simulink model "twoarea_system_test"  (R2014b)
settings: Solver=ode3  StartTime=0.0  StopTime=2  FixedStep=50e-6  RelTol=1e-3
libraries: powerlib x82
settings Model: Creator=saqibhasan  LastModifiedBy=saqibhasan
settings RTWCC: GenCodeOnly=on

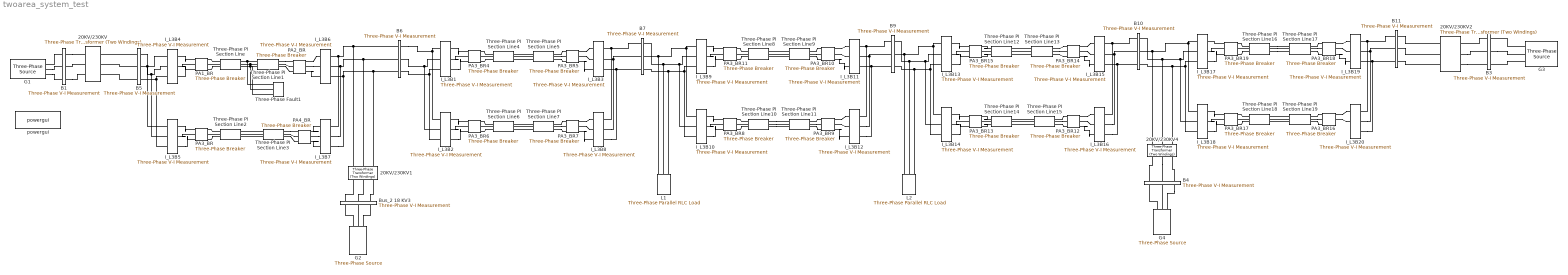
== system twoarea_system_test ==
  20KV/230KV : powerlib/Elements/Three-Phase Transformer (Two Windings)  Winding1Connection=Yg  UNITS=pu  NominalPower=[ 100e6 , 60 ]  Winding1=[ 20e3 , 0 , 3.980e-4]  Winding2Connection=Yg  Winding2=[ 230e3 , 0, 3.980e-4]  SetSaturation=off  Rm=500  Lm=500  Saturation=[ 0,0 ; 0.0024,1.2 ; 1.0,1.52 ]  Hysteresis=off  DataFile='hysteresis'  SetInitialFlux=off  InitialFluxes=[ 0.8 , -0.8 , 0.7 ]  Measurements=None  MoreParameters=off  BreakLoop=off  DataType=off  TransfoNumber=1
  20KV/230KV1 : powerlib/Elements/Three-Phase Transformer (Two Windings)  Winding1Connection=Yg  UNITS=pu  NominalPower=[ 900e6 , 60 ]  Winding1=[ 20e3 , 0 , 3.980e-4]  Winding2Connection=Yg  Winding2=[ 230e3 , 0, 3.980e-4]  SetSaturation=off  Rm=500  Lm=500  Saturation=[ 0,0 ; 0.0024,1.2 ; 1.0,1.52 ]  Hysteresis=off  DataFile='hysteresis'  SetInitialFlux=off  InitialFluxes=[ 0.8 , -0.8 , 0.7 ]  Measurements=None  MoreParameters=off  BreakLoop=off  DataType=off  TransfoNumber=1
  20KV/230KV2 : powerlib/Elements/Three-Phase Transformer (Two Windings)  Winding1Connection=Yg  UNITS=pu  NominalPower=[ 900e6 , 60 ]  Winding1=[ 20e3 , 0 , 3.980e-4]  Winding2Connection=Yg  Winding2=[ 230e3 , 0, 3.980e-4]  SetSaturation=off  Rm=500  Lm=500  Saturation=[ 0,0 ; 0.0024,1.2 ; 1.0,1.52 ]  Hysteresis=off  DataFile='hysteresis'  SetInitialFlux=off  InitialFluxes=[ 0.8 , -0.8 , 0.7 ]  Measurements=None  MoreParameters=off  BreakLoop=off  DataType=off  TransfoNumber=1
  20KV/230KV4 : powerlib/Elements/Three-Phase Transformer (Two Windings)  Winding1Connection=Yg  UNITS=pu  NominalPower=[ 900e6 , 60 ]  Winding1=[ 20e3 , 0 , 3.980e-4]  Winding2Connection=Yg  Winding2=[ 230e3 , 0, 3.980e-4]  SetSaturation=off  Rm=500  Lm=500  Saturation=[ 0,0 ; 0.0024,1.2 ; 1.0,1.52 ]  Hysteresis=off  DataFile='hysteresis'  SetInitialFlux=off  InitialFluxes=[ 0.8 , -0.8 , 0.7 ]  Measurements=None  MoreParameters=off  BreakLoop=off  DataType=off  TransfoNumber=1
  B1 : powerlib/Measurements/Three-Phase V-I Measurement  VoltageMeasurement=no  SetLabelV=off  LabelV=Vabc_B1  Vpu=off  VpuLL=off  CurrentMeasurement=no  SetLabelI=off  LabelI=Iabc_21  Ipu=off  Pbase=100e6  Vbase=20e3  OutputType=Complex  PhasorSimulation=off  PSBequivalent=0
  B10 : powerlib/Measurements/Three-Phase V-I Measurement  VoltageMeasurement=no  SetLabelV=on  LabelV=VB10  Vpu=off  VpuLL=off  CurrentMeasurement=no  SetLabelI=on  LabelI=Iabc_22  Ipu=off  Pbase=100e6  Vbase=230e3  OutputType=Complex  PhasorSimulation=off  PSBequivalent=0
  B11 : powerlib/Measurements/Three-Phase V-I Measurement  VoltageMeasurement=no  SetLabelV=on  LabelV=VB11  Vpu=off  VpuLL=off  CurrentMeasurement=no  SetLabelI=on  LabelI=Iabc_24  Ipu=off  Pbase=100e6  Vbase=230e3  OutputType=Complex  PhasorSimulation=off  PSBequivalent=0
  B3 : powerlib/Measurements/Three-Phase V-I Measurement  VoltageMeasurement=no  SetLabelV=on  LabelV=Vabc_3  Vpu=off  VpuLL=off  CurrentMeasurement=no  SetLabelI=on  LabelI=Iabc_23  Ipu=off  Pbase=100e6  Vbase=20e3  OutputType=Complex  PhasorSimulation=off  PSBequivalent=0
  B4 : powerlib/Measurements/Three-Phase V-I Measurement  VoltageMeasurement=no  SetLabelV=on  LabelV=Vabc_4  Vpu=off  VpuLL=off  CurrentMeasurement=no  SetLabelI=on  LabelI=Iabc_4  Ipu=off  Pbase=100e6  Vbase=20e3  OutputType=Complex  PhasorSimulation=off  PSBequivalent=0
  B5 : powerlib/Measurements/Three-Phase V-I Measurement  VoltageMeasurement=no  SetLabelV=on  LabelV=VB5  Vpu=off  VpuLL=off  CurrentMeasurement=no  SetLabelI=off  LabelI=Iabc_2  Ipu=off  Pbase=100e6  Vbase=230e3  OutputType=Complex  PhasorSimulation=off  PSBequivalent=0
  B6 : powerlib/Measurements/Three-Phase V-I Measurement  VoltageMeasurement=no  SetLabelV=on  LabelV=VB6  Vpu=off  VpuLL=off  CurrentMeasurement=no  SetLabelI=off  LabelI=Iabc_2  Ipu=off  Pbase=100e6  Vbase=230e3  OutputType=Complex  PhasorSimulation=off  PSBequivalent=0
  B7 : powerlib/Measurements/Three-Phase V-I Measurement  VoltageMeasurement=no  SetLabelV=on  LabelV=VB7  Vpu=off  VpuLL=off  CurrentMeasurement=no  SetLabelI=off  LabelI=Iabc_27  Ipu=off  Pbase=100e6  Vbase=230e3  OutputType=Complex  PhasorSimulation=off  PSBequivalent=0
  B9 : powerlib/Measurements/Three-Phase V-I Measurement  VoltageMeasurement=no  SetLabelV=on  LabelV=VB9  Vpu=off  VpuLL=off  CurrentMeasurement=no  SetLabelI=off  LabelI=Iabc_29  Ipu=off  Pbase=100e6  Vbase=230e3  OutputType=Complex  PhasorSimulation=off  PSBequivalent=0
  Bus_2 18 KV3 : powerlib/Measurements/Three-Phase V-I Measurement  VoltageMeasurement=no  SetLabelV=on  LabelV=Vabc_2  Vpu=off  VpuLL=off  CurrentMeasurement=no  SetLabelI=off  LabelI=Iabc_2  Ipu=off  Pbase=100e6  Vbase=20e3  OutputType=Complex  PhasorSimulation=off  PSBequivalent=0
  G1 : powerlib/Electrical Sources/Three-Phase Source  Voltage=20e3  PhaseAngle=0  Frequency=60  InternalConnection=Yg  SpecifyImpedance=on  Resistance=0.8929  Inductance=16.58e-3  ShortCircuitLevel=900e6  BaseVoltage=20e3  XRratio=10000  BusType=PV  Pref=900e6  Qref=144e6  Qmin=-inf  Qmax=600e6
  G2 : powerlib/Electrical Sources/Three-Phase Source  Voltage=20e3  PhaseAngle=0  Frequency=60  InternalConnection=Yg  SpecifyImpedance=on  Resistance=0.8929  Inductance=16.58e-3  ShortCircuitLevel=900e6  BaseVoltage=20e3  XRratio=10000  BusType=PV  Pref=900e6  Qref=300e6  Qmin=-inf  Qmax=300e6
  G3 : powerlib/Electrical Sources/Three-Phase Source  Voltage=20e3  PhaseAngle=0  Frequency=60  InternalConnection=Yg  SpecifyImpedance=on  Resistance=0.8929  Inductance=16.58e-3  ShortCircuitLevel=900e6  BaseVoltage=20e3  XRratio=100000  BusType=PV  Pref=900e6  Qref=-100e6  Qmin=-900e6  Qmax=-100e6
  G4 : powerlib/Electrical Sources/Three-Phase Source  Voltage=20e3  PhaseAngle=0  Frequency=60  InternalConnection=Yg  SpecifyImpedance=on  Resistance=0.8929  Inductance=16.58e-3  ShortCircuitLevel=900e6  BaseVoltage=20e3  XRratio=100000  BusType=PV  Pref=900e6  Qref=550e6  Qmin=-inf  Qmax=550e6
  I_L3B1 : powerlib/Measurements/Three-Phase V-I Measurement  VoltageMeasurement=no  SetLabelV=off  LabelV=Vabc  Vpu=off  VpuLL=off  CurrentMeasurement=no  SetLabelI=on  LabelI=IL21_22  Ipu=off  Pbase=100e6  Vbase=500e3  OutputType=Complex  PhasorSimulation=off  PSBequivalent=0
  I_L3B10 : powerlib/Measurements/Three-Phase V-I Measurement  VoltageMeasurement=no  SetLabelV=off  LabelV=Vabc  Vpu=off  VpuLL=off  CurrentMeasurement=no  SetLabelI=on  LabelI=IL33_34  Ipu=off  Pbase=100e6  Vbase=500e3  OutputType=Complex  PhasorSimulation=off  PSBequivalent=0
  I_L3B11 : powerlib/Measurements/Three-Phase V-I Measurement  VoltageMeasurement=no  SetLabelV=off  LabelV=Vabc  Vpu=off  VpuLL=off  CurrentMeasurement=no  SetLabelI=on  LabelI=IL32_31  Ipu=off  Pbase=100e6  Vbase=500e3  OutputType=Complex  PhasorSimulation=off  PSBequivalent=0
  I_L3B12 : powerlib/Measurements/Three-Phase V-I Measurement  VoltageMeasurement=no  SetLabelV=off  LabelV=Vabc  Vpu=off  VpuLL=off  CurrentMeasurement=no  SetLabelI=on  LabelI=IL34_33  Ipu=off  Pbase=100e6  Vbase=500e3  OutputType=Complex  PhasorSimulation=off  PSBequivalent=0
  I_L3B13 : powerlib/Measurements/Three-Phase V-I Measurement  VoltageMeasurement=no  SetLabelV=off  LabelV=Vabc  Vpu=off  VpuLL=off  CurrentMeasurement=no  SetLabelI=on  LabelI=IL41_42  Ipu=off  Pbase=100e6  Vbase=500e3  OutputType=Complex  PhasorSimulation=off  PSBequivalent=0
  I_L3B14 : powerlib/Measurements/Three-Phase V-I Measurement  VoltageMeasurement=no  SetLabelV=off  LabelV=Vabc  Vpu=off  VpuLL=off  CurrentMeasurement=no  SetLabelI=on  LabelI=IL43_44  Ipu=off  Pbase=100e6  Vbase=500e3  OutputType=Complex  PhasorSimulation=off  PSBequivalent=0
  I_L3B15 : powerlib/Measurements/Three-Phase V-I Measurement  VoltageMeasurement=no  SetLabelV=off  LabelV=Vabc  Vpu=off  VpuLL=off  CurrentMeasurement=no  SetLabelI=on  LabelI=IL42_41  Ipu=off  Pbase=100e6  Vbase=500e3  OutputType=Complex  PhasorSimulation=off  PSBequivalent=0
  I_L3B16 : powerlib/Measurements/Three-Phase V-I Measurement  VoltageMeasurement=no  SetLabelV=off  LabelV=Vabc  Vpu=off  VpuLL=off  CurrentMeasurement=no  SetLabelI=on  LabelI=IL44_43  Ipu=off  Pbase=100e6  Vbase=500e3  OutputType=Complex  PhasorSimulation=off  PSBequivalent=0
  I_L3B17 : powerlib/Measurements/Three-Phase V-I Measurement  VoltageMeasurement=no  SetLabelV=off  LabelV=Vabc  Vpu=off  VpuLL=off  CurrentMeasurement=no  SetLabelI=on  LabelI=IL51_52  Ipu=off  Pbase=100e6  Vbase=500e3  OutputType=Complex  PhasorSimulation=off  PSBequivalent=0
  I_L3B18 : powerlib/Measurements/Three-Phase V-I Measurement  VoltageMeasurement=no  SetLabelV=off  LabelV=Vabc  Vpu=off  VpuLL=off  CurrentMeasurement=no  SetLabelI=on  LabelI=IL53_54  Ipu=off  Pbase=100e6  Vbase=500e3  OutputType=Complex  PhasorSimulation=off  PSBequivalent=0
  I_L3B19 : powerlib/Measurements/Three-Phase V-I Measurement  VoltageMeasurement=no  SetLabelV=off  LabelV=Vabc  Vpu=off  VpuLL=off  CurrentMeasurement=no  SetLabelI=on  LabelI=IL52_51  Ipu=off  Pbase=100e6  Vbase=500e3  OutputType=Complex  PhasorSimulation=off  PSBequivalent=0
  I_L3B2 : powerlib/Measurements/Three-Phase V-I Measurement  VoltageMeasurement=no  SetLabelV=off  LabelV=Vabc  Vpu=off  VpuLL=off  CurrentMeasurement=no  SetLabelI=off  LabelI=IL23_24  Ipu=off  Pbase=100e6  Vbase=500e3  OutputType=Complex  PhasorSimulation=off  PSBequivalent=0
  I_L3B20 : powerlib/Measurements/Three-Phase V-I Measurement  VoltageMeasurement=no  SetLabelV=off  LabelV=Vabc  Vpu=off  VpuLL=off  CurrentMeasurement=no  SetLabelI=on  LabelI=IL54_53  Ipu=off  Pbase=100e6  Vbase=500e3  OutputType=Complex  PhasorSimulation=off  PSBequivalent=0
  I_L3B3 : powerlib/Measurements/Three-Phase V-I Measurement  VoltageMeasurement=no  SetLabelV=off  LabelV=Vabc  Vpu=off  VpuLL=off  CurrentMeasurement=no  SetLabelI=on  LabelI=IL22_21  Ipu=off  Pbase=100e6  Vbase=500e3  OutputType=Complex  PhasorSimulation=off  PSBequivalent=0
  I_L3B4 : powerlib/Measurements/Three-Phase V-I Measurement  VoltageMeasurement=no  SetLabelV=off  LabelV=Vabc  Vpu=off  VpuLL=off  CurrentMeasurement=no  SetLabelI=on  LabelI=IL11_12  Ipu=off  Pbase=100e6  Vbase=500e3  OutputType=Complex  PhasorSimulation=off  PSBequivalent=0
  I_L3B5 : powerlib/Measurements/Three-Phase V-I Measurement  VoltageMeasurement=no  SetLabelV=off  LabelV=Vabc  Vpu=off  VpuLL=off  CurrentMeasurement=no  SetLabelI=on  LabelI=IL13_14  Ipu=off  Pbase=100e6  Vbase=500e3  OutputType=Complex  PhasorSimulation=off  PSBequivalent=0
  I_L3B6 : powerlib/Measurements/Three-Phase V-I Measurement  VoltageMeasurement=no  SetLabelV=off  LabelV=Vabc  Vpu=off  VpuLL=off  CurrentMeasurement=no  SetLabelI=on  LabelI=IL12_11  Ipu=off  Pbase=100e6  Vbase=500e3  OutputType=Complex  PhasorSimulation=off  PSBequivalent=0
  I_L3B7 : powerlib/Measurements/Three-Phase V-I Measurement  VoltageMeasurement=no  SetLabelV=off  LabelV=Vabc  Vpu=off  VpuLL=off  CurrentMeasurement=no  SetLabelI=on  LabelI=IL14_13  Ipu=off  Pbase=100e6  Vbase=500e3  OutputType=Complex  PhasorSimulation=off  PSBequivalent=0
  I_L3B8 : powerlib/Measurements/Three-Phase V-I Measurement  VoltageMeasurement=no  SetLabelV=off  LabelV=Vabc  Vpu=off  VpuLL=off  CurrentMeasurement=no  SetLabelI=on  LabelI=IL24_23  Ipu=off  Pbase=100e6  Vbase=500e3  OutputType=Complex  PhasorSimulation=off  PSBequivalent=0
  I_L3B9 : powerlib/Measurements/Three-Phase V-I Measurement  VoltageMeasurement=no  SetLabelV=off  LabelV=Vabc  Vpu=off  VpuLL=off  CurrentMeasurement=no  SetLabelI=on  LabelI=IL31_32  Ipu=off  Pbase=100e6  Vbase=500e3  OutputType=Complex  PhasorSimulation=off  PSBequivalent=0
  L1 : powerlib/Elements/Three-Phase Parallel RLC Load  LConnTagsString=A|B|C  Configuration=Y (grounded)  NominalVoltage=230e3  NominalFrequency=60  ActivePower=967e6  InductivePower=100e6  CapacitivePower=200e6  Measurements=None  LoadType=constant PQ
  L2 : powerlib/Elements/Three-Phase Parallel RLC Load  LConnTagsString=A|B|C  Configuration=Y (grounded)  NominalVoltage=230e3  NominalFrequency=60  ActivePower=1767e6  InductivePower=100e6  CapacitivePower=350e6  Measurements=None  LoadType=constant PQ
  PA1_BR : powerlib/Elements/Three-Phase Breaker  InitialState=closed  SwitchA=on  SwitchB=on  SwitchC=on  SwitchTimes=[10]  External=off  BreakerResistance=1e-6  SnubberResistance=1e6  SnubberCapacitance=inf  Measurements=Breaker voltages and currents
  PA2_BR : powerlib/Elements/Three-Phase Breaker  InitialState=closed  SwitchA=on  SwitchB=on  SwitchC=on  SwitchTimes=[10]  External=off  BreakerResistance=1e-6  SnubberResistance=1e6  SnubberCapacitance=inf  Measurements=Breaker voltages and currents
  PA3_BR{,4..19} (17 alike) : powerlib/Elements/Three-Phase Breaker  InitialState=closed  SwitchA=on  SwitchB=on  SwitchC=on  SwitchTimes=[10]  External=off  BreakerResistance=1e-6  SnubberResistance=1e6  SnubberCapacitance=inf  Measurements=Breaker voltages and currents
  PA4_BR : powerlib/Elements/Three-Phase Breaker  InitialState=closed  SwitchA=on  SwitchB=on  SwitchC=on  SwitchTimes=[20]  External=off  BreakerResistance=1e-6  SnubberResistance=1e6  SnubberCapacitance=inf  Measurements=Breaker voltages and currents
  Three-Phase PI Section Line{,1..3,16..19} (8 alike) : powerlib/Elements/Three-Phase PI Section Line  LConnTagsString=a|b|c  RConnTagsString=A|B|C  Frequency=60  Resistances=[0.0529 0.1587]  Inductances="[.001404  .004212]"  Capacitances=[8.779e-9 26.339e-9]  Length=25
  Three-Phase PI Section Line{8..11} (4 alike) : powerlib/Elements/Three-Phase PI Section Line  LConnTagsString=a|b|c  RConnTagsString=A|B|C  Frequency=60  Resistances=[0.0529 0.1587]  Inductances="[.001404  .004212]"  Capacitances=[8.779e-9 26.339e-9]  Length=220
  Three-Phase PI Section Line{4..7,12..15} (8 alike) : powerlib/Elements/Three-Phase PI Section Line  LConnTagsString=a|b|c  RConnTagsString=A|B|C  Frequency=60  Resistances=[0.0529 0.1587]  Inductances="[.001404  .004212]"  Capacitances=[8.779e-9 26.339e-9]  Length=10
  Three-Phase Fault1 : powerlib/Elements/Three-Phase Fault  InitialStates=0  FaultA=on  FaultB=on  FaultC=on  GroundFault=on  SwitchTimes=[11]  External=off  SwitchStatus=NaN  FaultResistance=0.001  GroundResistance=0.01  SnubberResistance=1e6  SnubberCapacitance=inf  Measurements=None
  powergui : powerlib/powergui  Priority=1  SimulationMode=Discrete  SolverType=Tustin  SampleTime=50e-6  frequency=60  SPID=on  DisableSnubberDevices=off  DisableRonSwitches=off  DisableVfSwitches=off  SwTol=0  DisplayEquations=off  Interpol=off  methode=off  Ts=0  frequencyindice=60  Pbase=10e7  ErrMax=1e-05  Iterations=50  UnitsV=kV  UnitsW=MW  FunctionMessages=off  echomessages=off  HookPort=off  EnableUseOfTLC=off  x0status=blocks  RestoreLinks=warning  ResistiveCurrentMeasurement=off  Frange=[0:2:500]  Ylog=off  Xlog=on  ShowGrid=off  save=off  variable=ZData  structure=0  ZoomFFT=off  StartTime=0.0  cycles=1  DisplayStyle=1  fundamental=60  FreqAxis=off  MaxFrequency=1000  frequencyindicesteady=1  RmsSteady=1  display=off
  connections:
  B5/LConn1 -- 20KV/230KV/RConn1
  B5/LConn2 -- 20KV/230KV/RConn2
  B5/LConn3 -- 20KV/230KV/RConn3
  B1/RConn1 -- 20KV/230KV/LConn1
  B1/RConn2 -- 20KV/230KV/LConn2
  B1/RConn3 -- 20KV/230KV/LConn3
  B1/LConn1 -- G1/RConn1
  G1/RConn2 -- B1/LConn2
  G1/RConn3 -- B1/LConn3
  B3/LConn2 -- G3/RConn2
  G3/RConn1 -- B3/LConn1
  G3/RConn3 -- B3/LConn3
  20KV/230KV2/LConn2 -- B3/RConn2
  20KV/230KV2/LConn3 -- B3/RConn3
  B4/LConn3 -- G4/RConn3
  G4/RConn2 -- B4/LConn2
  G4/RConn1 -- B4/LConn1
  20KV/230KV4/LConn2 -- B4/RConn2
  B4/RConn3 -- 20KV/230KV4/LConn3
  B3/RConn1 -- 20KV/230KV2/LConn1
  B4/RConn1 -- 20KV/230KV4/LConn1
  I_L3B4/LConn3 -- I_L3B5/LConn3 -- B5/RConn3
  B5/RConn2 -- I_L3B4/LConn2 -- I_L3B5/LConn2
  B5/RConn1 -- I_L3B5/LConn1 -- I_L3B4/LConn1
  I_L3B6/LConn2 -- 20KV/230KV1/RConn2 -- B6/LConn2 -- I_L3B7/LConn2
  I_L3B6/LConn1 -- I_L3B7/LConn1 -- 20KV/230KV1/RConn1 -- B6/LConn1
  I_L3B6/LConn3 -- 20KV/230KV1/RConn3 -- B6/LConn3 -- I_L3B7/LConn3
  G2/RConn1 -- Bus_2 18 KV3/LConn1
  G2/RConn2 -- Bus_2 18 KV3/LConn2
  G2/RConn3 -- Bus_2 18 KV3/LConn3
  Bus_2 18 KV3/RConn1 -- 20KV/230KV1/LConn1
  Bus_2 18 KV3/RConn2 -- 20KV/230KV1/LConn2
  Bus_2 18 KV3/RConn3 -- 20KV/230KV1/LConn3
  Three-Phase Fault1/LConn1 -- Three-Phase PI Section Line1/LConn1 -- Three-Phase PI Section Line/RConn1
  Three-Phase Fault1/LConn2 -- Three-Phase PI Section Line1/LConn2 -- Three-Phase PI Section Line/RConn2
  Three-Phase Fault1/LConn3 -- Three-Phase PI Section Line1/LConn3 -- Three-Phase PI Section Line/RConn3
  Three-Phase PI Section Line3/LConn3 -- Three-Phase PI Section Line2/RConn3
  Three-Phase PI Section Line3/LConn1 -- Three-Phase PI Section Line2/RConn1
  Three-Phase PI Section Line3/LConn2 -- Three-Phase PI Section Line2/RConn2
  I_L3B1/LConn3 -- B6/RConn3 -- I_L3B2/LConn3
  I_L3B2/LConn2 -- I_L3B1/LConn2 -- B6/RConn2
  I_L3B3/LConn2 -- B7/LConn2 -- I_L3B8/LConn2
  I_L3B3/LConn1 -- B7/LConn1 -- I_L3B8/LConn1
  I_L3B3/LConn3 -- B7/LConn3 -- I_L3B8/LConn3
  Three-Phase PI Section Line5/LConn2 -- Three-Phase PI Section Line4/RConn2
  Three-Phase PI Section Line5/LConn3 -- Three-Phase PI Section Line4/RConn3
  Three-Phase PI Section Line5/LConn1 -- Three-Phase PI Section Line4/RConn1
  Three-Phase PI Section Line7/LConn1 -- Three-Phase PI Section Line6/RConn1
  Three-Phase PI Section Line7/LConn2 -- Three-Phase PI Section Line6/RConn2
  Three-Phase PI Section Line7/LConn3 -- Three-Phase PI Section Line6/RConn3
  B6/RConn1 -- I_L3B2/LConn1 -- I_L3B1/LConn1
  I_L3B9/LConn3 -- B7/RConn3 -- L1/LConn3 -- I_L3B10/LConn3
  I_L3B10/LConn2 -- B7/RConn2 -- L1/LConn2 -- I_L3B9/LConn2
  I_L3B11/LConn2 -- B9/LConn2 -- I_L3B12/LConn2
  I_L3B11/LConn1 -- B9/LConn1 -- I_L3B12/LConn1
  I_L3B11/LConn3 -- B9/LConn3 -- I_L3B12/LConn3
  Three-Phase PI Section Line9/LConn1 -- Three-Phase PI Section Line8/RConn1
  Three-Phase PI Section Line10/RConn1 -- Three-Phase PI Section Line11/LConn1
  Three-Phase PI Section Line9/LConn3 -- Three-Phase PI Section Line8/RConn3
  Three-Phase PI Section Line9/LConn2 -- Three-Phase PI Section Line8/RConn2
  Three-Phase PI Section Line10/RConn3 -- Three-Phase PI Section Line11/LConn3
  Three-Phase PI Section Line10/RConn2 -- Three-Phase PI Section Line11/LConn2
  I_L3B9/LConn1 -- I_L3B10/LConn1 -- B7/RConn1 -- L1/LConn1
  I_L3B13/LConn3 -- L2/LConn3 -- B9/RConn3 -- I_L3B14/LConn3
  I_L3B14/LConn2 -- L2/LConn2 -- B9/RConn2 -- I_L3B13/LConn2
  I_L3B15/LConn2 -- B10/LConn2 -- I_L3B16/LConn2
  I_L3B15/LConn1 -- B10/LConn1 -- I_L3B16/LConn1
  I_L3B15/LConn3 -- B10/LConn3 -- I_L3B16/LConn3
  Three-Phase PI Section Line13/LConn1 -- Three-Phase PI Section Line12/RConn1
  Three-Phase PI Section Line15/LConn1 -- Three-Phase PI Section Line14/RConn1
  Three-Phase PI Section Line13/LConn3 -- Three-Phase PI Section Line12/RConn3
  Three-Phase PI Section Line13/LConn2 -- Three-Phase PI Section Line12/RConn2
  Three-Phase PI Section Line15/LConn3 -- Three-Phase PI Section Line14/RConn3
  Three-Phase PI Section Line15/LConn2 -- Three-Phase PI Section Line14/RConn2
  I_L3B13/LConn1 -- L2/LConn1 -- B9/RConn1 -- I_L3B14/LConn1
  I_L3B17/LConn3 -- B10/RConn3 -- 20KV/230KV4/RConn3 -- I_L3B18/LConn3
  I_L3B18/LConn2 -- B10/RConn2 -- 20KV/230KV4/RConn2 -- I_L3B17/LConn2
  I_L3B19/LConn2 -- B11/LConn2 -- I_L3B20/LConn2
  I_L3B19/LConn1 -- B11/LConn1 -- I_L3B20/LConn1
  I_L3B19/LConn3 -- B11/LConn3 -- I_L3B20/LConn3
  Three-Phase PI Section Line19/LConn3 -- Three-Phase PI Section Line18/RConn3
  Three-Phase PI Section Line19/LConn2 -- Three-Phase PI Section Line18/RConn2
  I_L3B17/LConn1 -- 20KV/230KV4/RConn1 -- B10/RConn1 -- I_L3B18/LConn1
  Three-Phase PI Section Line16/RConn1 -- Three-Phase PI Section Line17/LConn1
  Three-Phase PI Section Line19/LConn1 -- Three-Phase PI Section Line18/RConn1
  Three-Phase PI Section Line16/RConn3 -- Three-Phase PI Section Line17/LConn3
  Three-Phase PI Section Line16/RConn2 -- Three-Phase PI Section Line17/LConn2
  B11/RConn1 -- 20KV/230KV2/RConn1
  B11/RConn2 -- 20KV/230KV2/RConn2
  B11/RConn3 -- 20KV/230KV2/RConn3
  Three-Phase PI Section Line/LConn1 -- PA1_BR/RConn1
  Three-Phase PI Section Line/LConn2 -- PA1_BR/RConn2
  Three-Phase PI Section Line/LConn3 -- PA1_BR/RConn3
  I_L3B4/RConn1 -- PA1_BR/LConn1
  I_L3B4/RConn2 -- PA1_BR/LConn2
  I_L3B4/RConn3 -- PA1_BR/LConn3
  Three-Phase PI Section Line1/RConn1 -- PA2_BR/LConn1
  Three-Phase PI Section Line1/RConn2 -- PA2_BR/LConn2
  Three-Phase PI Section Line1/RConn3 -- PA2_BR/LConn3
  PA2_BR/RConn1 -- I_L3B6/RConn1
  PA2_BR/RConn2 -- I_L3B6/RConn2
  PA2_BR/RConn3 -- I_L3B6/RConn3
  Three-Phase PI Section Line2/LConn1 -- PA3_BR/RConn1
  Three-Phase PI Section Line2/LConn2 -- PA3_BR/RConn2
  Three-Phase PI Section Line2/LConn3 -- PA3_BR/RConn3
  I_L3B5/RConn1 -- PA3_BR/LConn1
  I_L3B5/RConn2 -- PA3_BR/LConn2
  I_L3B5/RConn3 -- PA3_BR/LConn3
  Three-Phase PI Section Line3/RConn1 -- PA4_BR/LConn1
  Three-Phase PI Section Line3/RConn2 -- PA4_BR/LConn2
  Three-Phase PI Section Line3/RConn3 -- PA4_BR/LConn3
  PA4_BR/RConn1 -- I_L3B7/RConn1
  PA4_BR/RConn2 -- I_L3B7/RConn2
  PA4_BR/RConn3 -- I_L3B7/RConn3
  Three-Phase PI Section Line4/LConn1 -- PA3_BR4/RConn1
  Three-Phase PI Section Line4/LConn2 -- PA3_BR4/RConn2
  Three-Phase PI Section Line4/LConn3 -- PA3_BR4/RConn3
  I_L3B1/RConn1 -- PA3_BR4/LConn1
  I_L3B1/RConn2 -- PA3_BR4/LConn2
  I_L3B1/RConn3 -- PA3_BR4/LConn3
  PA3_BR5/RConn1 -- I_L3B3/RConn1
  Three-Phase PI Section Line5/RConn1 -- PA3_BR5/LConn1
  Three-Phase PI Section Line5/RConn2 -- PA3_BR5/LConn2
  Three-Phase PI Section Line5/RConn3 -- PA3_BR5/LConn3
  PA3_BR5/RConn2 -- I_L3B3/RConn2
  PA3_BR5/RConn3 -- I_L3B3/RConn3
  Three-Phase PI Section Line6/LConn1 -- PA3_BR6/RConn1
  Three-Phase PI Section Line6/LConn2 -- PA3_BR6/RConn2
  Three-Phase PI Section Line6/LConn3 -- PA3_BR6/RConn3
  I_L3B2/RConn1 -- PA3_BR6/LConn1
  I_L3B2/RConn2 -- PA3_BR6/LConn2
  I_L3B2/RConn3 -- PA3_BR6/LConn3
  Three-Phase PI Section Line7/RConn1 -- PA3_BR7/LConn1
  Three-Phase PI Section Line7/RConn2 -- PA3_BR7/LConn2
  Three-Phase PI Section Line7/RConn3 -- PA3_BR7/LConn3
  PA3_BR7/RConn1 -- I_L3B8/RConn1
  PA3_BR7/RConn2 -- I_L3B8/RConn2
  PA3_BR7/RConn3 -- I_L3B8/RConn3
  Three-Phase PI Section Line8/LConn1 -- PA3_BR11/RConn1
  Three-Phase PI Section Line8/LConn2 -- PA3_BR11/RConn2
  Three-Phase PI Section Line8/LConn3 -- PA3_BR11/RConn3
  I_L3B9/RConn1 -- PA3_BR11/LConn1
  I_L3B9/RConn2 -- PA3_BR11/LConn2
  I_L3B9/RConn3 -- PA3_BR11/LConn3
  Three-Phase PI Section Line9/RConn1 -- PA3_BR10/LConn1
  Three-Phase PI Section Line9/RConn2 -- PA3_BR10/LConn2
  Three-Phase PI Section Line9/RConn3 -- PA3_BR10/LConn3
  PA3_BR10/RConn1 -- I_L3B11/RConn1
  PA3_BR10/RConn2 -- I_L3B11/RConn2
  PA3_BR10/RConn3 -- I_L3B11/RConn3
  Three-Phase PI Section Line10/LConn1 -- PA3_BR8/RConn1
  Three-Phase PI Section Line10/LConn2 -- PA3_BR8/RConn2
  Three-Phase PI Section Line10/LConn3 -- PA3_BR8/RConn3
  I_L3B10/RConn1 -- PA3_BR8/LConn1
  I_L3B10/RConn2 -- PA3_BR8/LConn2
  I_L3B10/RConn3 -- PA3_BR8/LConn3
  Three-Phase PI Section Line11/RConn1 -- PA3_BR9/LConn1
  Three-Phase PI Section Line11/RConn2 -- PA3_BR9/LConn2
  Three-Phase PI Section Line11/RConn3 -- PA3_BR9/LConn3
  PA3_BR9/RConn1 -- I_L3B12/RConn1
  PA3_BR9/RConn2 -- I_L3B12/RConn2
  PA3_BR9/RConn3 -- I_L3B12/RConn3
  Three-Phase PI Section Line12/LConn1 -- PA3_BR15/RConn1
  Three-Phase PI Section Line12/LConn2 -- PA3_BR15/RConn2
  Three-Phase PI Section Line12/LConn3 -- PA3_BR15/RConn3
  I_L3B13/RConn1 -- PA3_BR15/LConn1
  I_L3B13/RConn2 -- PA3_BR15/LConn2
  I_L3B13/RConn3 -- PA3_BR15/LConn3
  PA3_BR14/RConn1 -- I_L3B15/RConn1
  Three-Phase PI Section Line13/RConn1 -- PA3_BR14/LConn1
  Three-Phase PI Section Line13/RConn2 -- PA3_BR14/LConn2
  Three-Phase PI Section Line13/RConn3 -- PA3_BR14/LConn3
  PA3_BR14/RConn2 -- I_L3B15/RConn2
  PA3_BR14/RConn3 -- I_L3B15/RConn3
  Three-Phase PI Section Line14/LConn1 -- PA3_BR13/RConn1
  Three-Phase PI Section Line14/LConn2 -- PA3_BR13/RConn2
  Three-Phase PI Section Line14/LConn3 -- PA3_BR13/RConn3
  I_L3B14/RConn1 -- PA3_BR13/LConn1
  I_L3B14/RConn2 -- PA3_BR13/LConn2
  I_L3B14/RConn3 -- PA3_BR13/LConn3
  Three-Phase PI Section Line15/RConn1 -- PA3_BR12/LConn1
  Three-Phase PI Section Line15/RConn2 -- PA3_BR12/LConn2
  Three-Phase PI Section Line15/RConn3 -- PA3_BR12/LConn3
  PA3_BR12/RConn1 -- I_L3B16/RConn1
  PA3_BR12/RConn2 -- I_L3B16/RConn2
  PA3_BR12/RConn3 -- I_L3B16/RConn3
  Three-Phase PI Section Line16/LConn1 -- PA3_BR19/RConn1
  Three-Phase PI Section Line16/LConn2 -- PA3_BR19/RConn2
  Three-Phase PI Section Line16/LConn3 -- PA3_BR19/RConn3
  PA3_BR19/LConn1 -- I_L3B17/RConn1
  I_L3B17/RConn2 -- PA3_BR19/LConn2
  I_L3B17/RConn3 -- PA3_BR19/LConn3
  PA3_BR18/RConn1 -- I_L3B19/RConn1
  Three-Phase PI Section Line17/RConn1 -- PA3_BR18/LConn1
  Three-Phase PI Section Line17/RConn2 -- PA3_BR18/LConn2
  Three-Phase PI Section Line17/RConn3 -- PA3_BR18/LConn3
  PA3_BR18/RConn2 -- I_L3B19/RConn2
  PA3_BR18/RConn3 -- I_L3B19/RConn3
  Three-Phase PI Section Line18/LConn1 -- PA3_BR17/RConn1
  Three-Phase PI Section Line18/LConn2 -- PA3_BR17/RConn2
  Three-Phase PI Section Line18/LConn3 -- PA3_BR17/RConn3
  I_L3B18/RConn1 -- PA3_BR17/LConn1
  I_L3B18/RConn2 -- PA3_BR17/LConn2
  I_L3B18/RConn3 -- PA3_BR17/LConn3
  Three-Phase PI Section Line19/RConn1 -- PA3_BR16/LConn1
  Three-Phase PI Section Line19/RConn2 -- PA3_BR16/LConn2
  Three-Phase PI Section Line19/RConn3 -- PA3_BR16/LConn3
  PA3_BR16/RConn1 -- I_L3B20/RConn1
  PA3_BR16/RConn2 -- I_L3B20/RConn2
